simulink model "open_loop_hinf_3"  (R2025b)
settings: Solver=VariableStepAuto  StartTime=0.0  StopTime=10.0  RelTol=1e-3
undefined symbols (not defined in the file or in its folder): alpha, Den, eta_0, Js, Num, omega, taue, xi
settings Model: Creator=ruben  LastModifiedBy=ruben

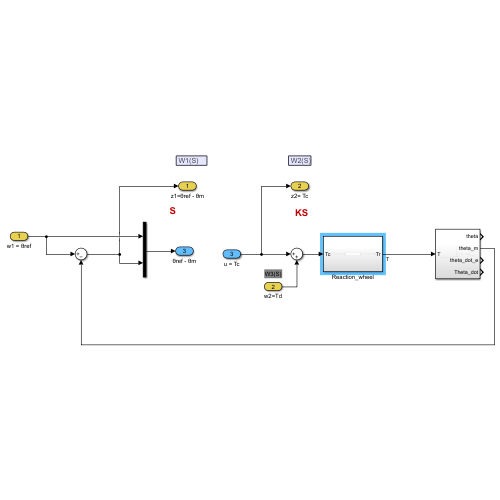
[thumbnail: Simulink's stored preview of the top-level diagram]
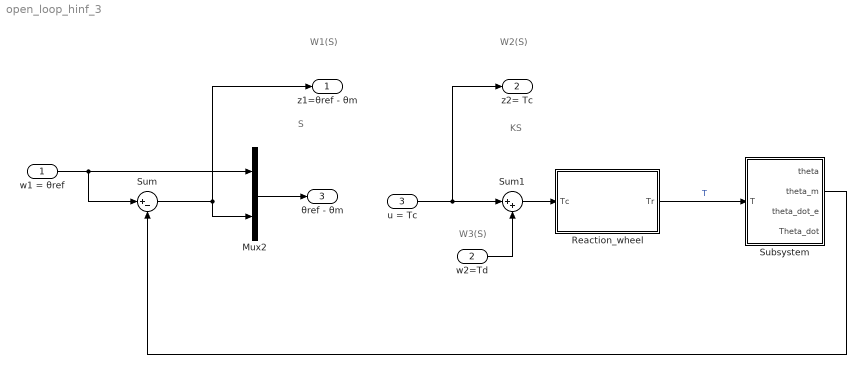
== system open_loop_hinf_3 ==
  note: W3(S)
  note: W2(S)
  note: KS
  note: W1(S)
  note: S
  w1 = θref : Inport
  w2=Td : Inport  Port=2
  u = Tc : Inport  Port=3
  Mux2 : Mux  Inputs=2
  Reaction_wheel : Subsystem
  Subsystem : Subsystem
  Sum : Sum  Inputs=|+-
  Sum1 : Sum  Inputs=|++
  z1=θref - θm : Outport
  z2= Tc : Outport  Port=2
  θref - θm : Outport  Port=3
  wires:
  Subsystem/2(theta_m) -> Sum/2
  u = Tc/1 -> Sum1/1, z2= Tc/1
  Reaction_wheel/1(Tr) -> Subsystem/1(T)  "T"
  w2=Td/1 -> Sum1/2
  Sum1/1 -> Reaction_wheel/1(Tc)
  Mux2/1 -> θref - θm/1
  Sum/1 -> z1=θref - θm/1, Mux2/2
  w1 = θref/1 -> Sum/1, Mux2/1

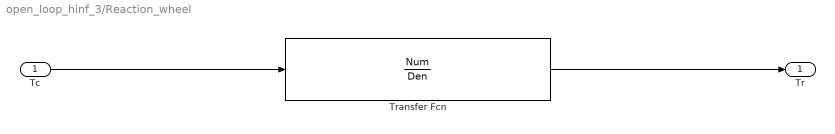
== system open_loop_hinf_3/Reaction_wheel ==
  Tc : Inport
  Transfer Fcn : TransferFcn  Numerator=Num  Denominator=Den
  Tr : Outport
  wires:
  Transfer Fcn/1 -> Tr/1
  Tc/1 -> Transfer Fcn/1

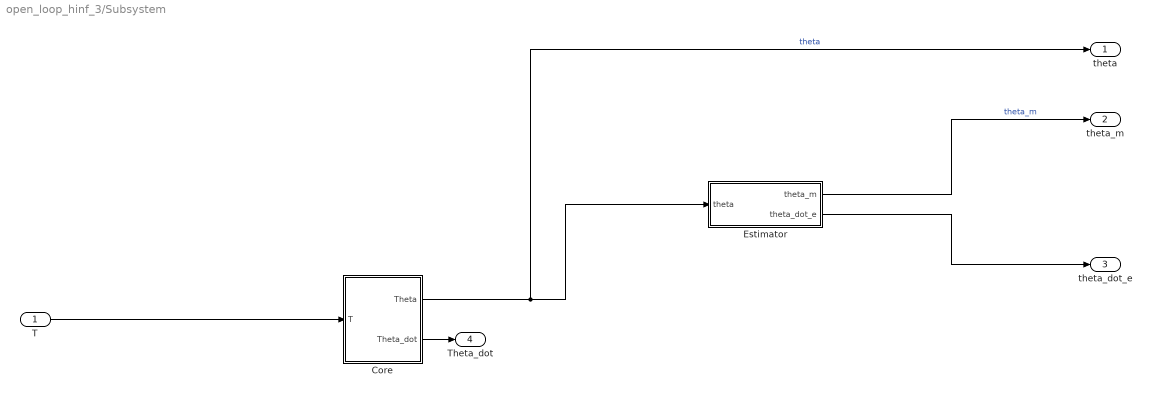
== system open_loop_hinf_3/Subsystem ==
  T : Inport
  Core : Subsystem
  Estimator : Subsystem
  theta : Outport
  theta_m : Outport  Port=2
  theta_dot_e : Outport  Port=3
  Theta_dot : Outport  Port=4
  wires:
  Core/1(Theta) -> theta/1, Estimator/1(theta)  "theta"
  Core/2(Theta_dot) -> Theta_dot/1
  Estimator/2(theta_dot_e) -> theta_dot_e/1
  Estimator/1(theta_m) -> theta_m/1  "theta_m"
  T/1 -> Core/1(T)

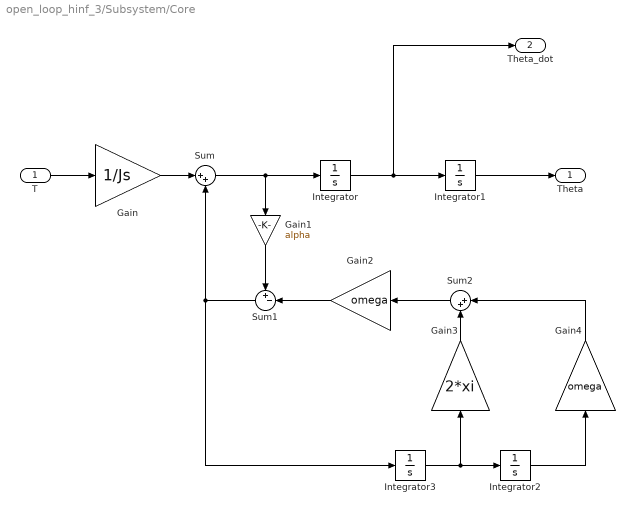
== system open_loop_hinf_3/Subsystem/Core ==
  T : Inport
  Gain : Gain  Gain=1/Js
  Gain1 : Gain  Gain=alpha
  Gain2 : Gain  Gain=omega
  Gain3 : Gain  Gain=2*xi
  Gain4 : Gain  Gain=omega
  Integrator : Integrator
  Integrator1 : Integrator
  Integrator2 : Integrator  InitialCondition=eta_0
  Integrator3 : Integrator
  Sum : Sum  Inputs=|++
  Sum1 : Sum  Inputs=+-|
  Sum2 : Sum  Inputs=|++
  Theta : Outport
  Theta_dot : Outport  Port=2
  wires:
  Integrator/1 -> Theta_dot/1, Integrator1/1
  Gain4/1 -> Sum2/1
  Sum/1 -> Gain1/1, Integrator/1
  Gain2/1 -> Sum1/2
  Sum1/1 -> Integrator3/1, Sum/2
  Gain1/1 -> Sum1/1
  Gain3/1 -> Sum2/2
  Integrator3/1 -> Integrator2/1, Gain3/1
  Sum2/1 -> Gain2/1
  T/1 -> Gain/1
  Integrator1/1 -> Theta/1
  Gain/1 -> Sum/1
  Integrator2/1 -> Gain4/1

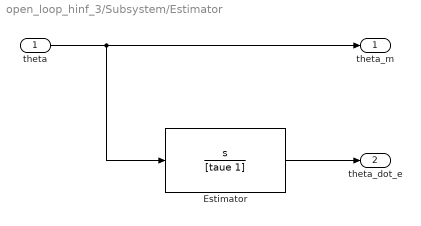
== system open_loop_hinf_3/Subsystem/Estimator ==
  theta : Inport
  Estimator : TransferFcn  Numerator=[1 0]  Denominator=[taue 1]
  theta_m : Outport
  theta_dot_e : Outport  Port=2
  wires:
  theta/1 -> theta_m/1, Estimator/1
  Estimator/1 -> theta_dot_e/1
